simulink model "sim_variable_structure1"  (R2020a)
settings: Solver=FixedStepAuto  StartTime=0.0  StopTime=end_time  FixedStep=FStep  RelTol=1e-3
undefined symbols (not defined in the file): b, c, K0, T1, T2
libraries: simulink_extras x3
settings Model: Creator=ogure  LastModifiedBy=my000
settings SolverCC: SolverResetMethod=Robust
settings DataIOCC: SaveFormat=Array  SaveOutput=off  SignalLogging=off  ReturnWorkspaceOutputs=off
settings DebuggingCC: SolverPrmCheckMsg=warning
settings SFSimCC: CustomCodeUndefinedFunction=UseInterfaceOnly

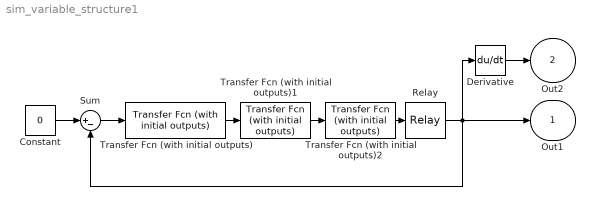
== system sim_variable_structure1 ==
  Constant : Constant  Value=0
  Derivative : Derivative
  Relay : Relay  OnSwitchValue=b  OffSwitchValue=-b  OnOutputValue=c  OffOutputValue=-c
  Sum : Sum  Inputs=|+-
  Transfer Fcn (with initial outputs) : simulink_extras/Additional Linear/Transfer Fcn (with initial outputs)  N=[K0]  D="[T1  1]"  Y0=y0  U0=0
  Transfer Fcn (with initial outputs)1 : simulink_extras/Additional Linear/Transfer Fcn (with initial outputs)  N=[1]  D="[T2  1]"  Y0=x0  U0=0
  Transfer Fcn (with initial outputs)2 : simulink_extras/Additional Linear/Transfer Fcn (with initial outputs)  N=[1]  D="[0.2  1]"  Y0=x0  U0=0
  Out1 : Outport  SignalName=x  VectorParamsAs1DForOutWhenUnconnected=off
  Out2 : Outport  Port=2  SignalName=y  VectorParamsAs1DForOutWhenUnconnected=off
  wires:
  Derivative/1 -> Out2/1
  Relay/1 -> Sum/2, Out1/1, Derivative/1
  Sum/1 -> Transfer Fcn (with initial outputs)/1
  Constant/1 -> Sum/1
  Transfer Fcn (with initial outputs)/1 -> Transfer Fcn (with initial outputs)1/1
  Transfer Fcn (with initial outputs)1/1 -> Transfer Fcn (with initial outputs)2/1
  Transfer Fcn (with initial outputs)2/1 -> Relay/1
